simulink model "switchTank"  (R2014b)
settings: Solver=FixedStepDiscrete  StartTime=0.0  StopTime=100000  FixedStep=0.01  MaxStep=0.0001  RelTol=1e-3
settings Model: Creator=sand080  LastModifiedBy=sand080
settings DataIOCC: LimitDataPoints=off

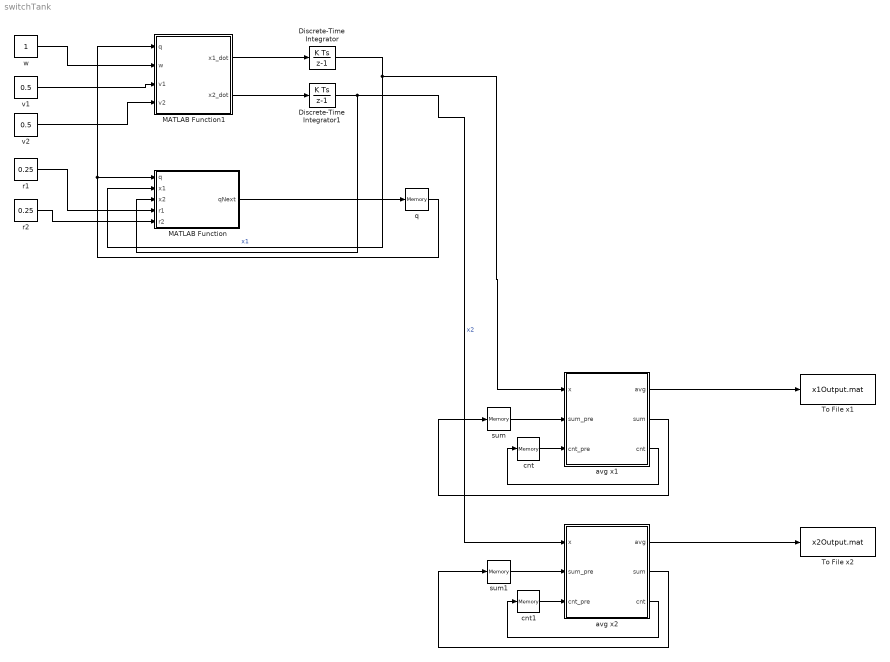
== system switchTank ==
  Discrete-Time Integrator : DiscreteIntegrator  InitialCondition=0.5  InitialConditionSetting=State (most efficient)  SampleTime=-1
  Discrete-Time Integrator1 : DiscreteIntegrator  InitialCondition=0.5  InitialConditionSetting=State (most efficient)  SampleTime=-1
  MATLAB Function : MATLAB Function  TreatAsAtomicUnit=on
  MATLAB Function1 : MATLAB Function  TreatAsAtomicUnit=on
  To File x1 : ToFile  Filename=x1Output.mat
      settings: Decimation=10000000
  To File x2 : ToFile  Filename=x2Output.mat
      settings: Decimation=10000000
  avg x1 : MATLAB Function  TreatAsAtomicUnit=on
  avg x2 : MATLAB Function  TreatAsAtomicUnit=on
  cnt : Memory
  cnt1 : Memory
  q : Memory  X0=1
  r1 : Constant  Value=0.25
  r2 : Constant  Value=0.25
  sum : Memory
  sum1 : Memory
  v1 : Constant  Value=0.5
  v2 : Constant  Value=0.5
  w : Constant
  wires:
  MATLAB Function/1(qNext) -> q/1
  MATLAB Function1/1(x1_dot) -> Discrete-Time Integrator/1
  MATLAB Function1/2(x2_dot) -> Discrete-Time Integrator1/1
  Discrete-Time Integrator/1 -> MATLAB Function/2(x1), avg x1/1(x)  "x1"
  q/1 -> MATLAB Function1/1(q), MATLAB Function/1(q)
  v1/1 -> MATLAB Function1/3(v1)
  v2/1 -> MATLAB Function1/4(v2)
  r1/1 -> MATLAB Function/4(r1)
  r2/1 -> MATLAB Function/5(r2)
  w/1 -> MATLAB Function1/2(w)
  Discrete-Time Integrator1/1 -> MATLAB Function/3(x2), avg x2/1(x)  "x2"
  avg x1/2(sum) -> sum/1
  avg x1/3(cnt) -> cnt/1
  cnt/1 -> avg x1/3(cnt_pre)
  sum/1 -> avg x1/2(sum_pre)
  avg x1/1(avg) -> To File x1/1
  avg x2/2(sum) -> sum1/1
  avg x2/3(cnt) -> cnt1/1
  cnt1/1 -> avg x2/3(cnt_pre)
  sum1/1 -> avg x2/2(sum_pre)
  avg x2/1(avg) -> To File x2/1

== matlab function switchTank/MATLAB Function1 ==
  data: q input; x1_dot output; w input; v1 input; v2 input; x2_dot output
function [x1_dot,x2_dot]= flow(q,w,v1,v2)
%#codegen
if q==1 
    x1_dot = w-v1;
    x2_dot = -v2;
else
    x1_dot = -v1;
    x2_dot = w-v2;
end

== matlab function switchTank/MATLAB Function ==
  data: q input; qNext output; x1 input; x2 input; r1 input; r2 input
function qNext = phi(q,x1,x2, r1, r2)
%#codegen
if q==1 && x2 < r2
    qNext=2;
elseif q==1 && x2 >= r2
    qNext=1;
elseif q==2 && x1 < r1
    qNext=1;
elseif q==2 && x1 >= r1
    qNext=2;
else
    qNext=0; %this should never execute
end

== matlab function switchTank/avg x1 ==
  data: x input; avg output; sum output; cnt output; sum_pre input; cnt_pre input
function [avg, sum,cnt] = fcn(x,  sum_pre, cnt_pre)
%#codegen

cnt=cnt_pre+1;
sum=sum_pre+x;
avg=sum/cnt;

== matlab function switchTank/avg x2 ==
  data: x input; avg output; sum output; cnt output; sum_pre input; cnt_pre input
function [avg, sum,cnt] = fcn(x,  sum_pre, cnt_pre)
%#codegen

cnt=cnt_pre+1;
sum=sum_pre+x;
avg=sum/cnt;
